simulink model "PID_Continous_Discrete"  (R2024a)
settings: Solver=FixedStepDiscrete  StartTime=0.0  StopTime=10.0  FixedStep=1e-3  RelTol=1e-3
libraries: simulink x1
settings Model: Creator=VICTUS  LastModifiedBy=VICTUS

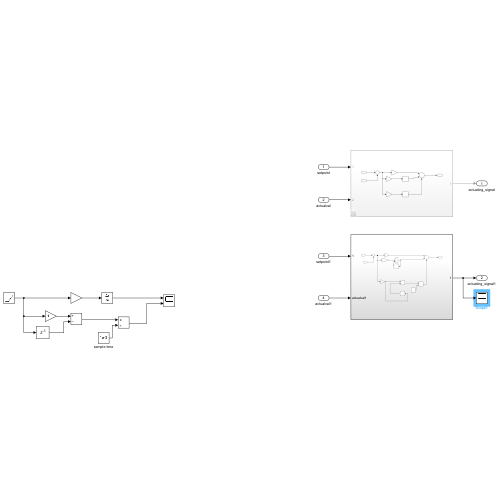
[thumbnail: Simulink's stored preview of the top-level diagram]
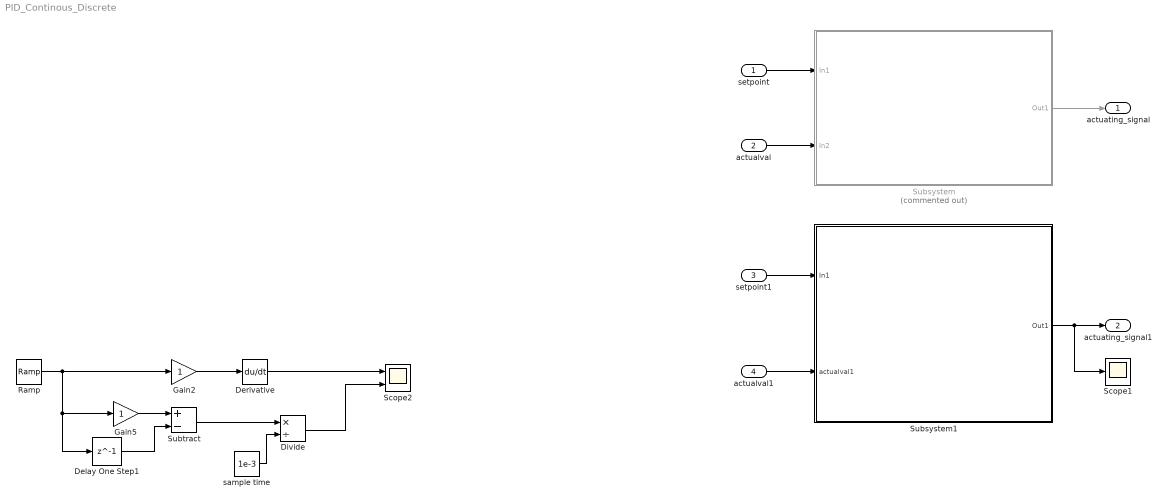
== system PID_Continous_Discrete ==
  setpoint : Inport
  actualval : Inport  Port=2
  setpoint1 : Inport  Port=3
  actualval1 : Inport  Port=4
  Delay One Step1 : Delay  DelayLength=1
  Derivative : Derivative  CoefficientInTFapproximation=1/(1e-3)
  Divide : Product  Inputs=*/
  Gain2 : Gain
  Gain5 : Gain
  Ramp : simulink/Sources/Ramp  slope=1  start=0  InitialOutput=0
  Scope1 : Scope
  Scope2 : Scope  NumInputPorts=2
  Subsystem : Subsystem  Commented=on
  Subsystem1 : Subsystem
  Subtract : Sum  Inputs=+-
  sample time : Constant  Value=1e-3
  actuating_signal : Outport
  actuating_signal1 : Outport  Port=2
  wires:
  Subsystem/1(Out1) -> actuating_signal/1
  Subsystem1/1(Out1) -> Scope1/1, actuating_signal1/1
  setpoint/1 -> Subsystem/1(In1)
  actualval/1 -> Subsystem/2(In2)
  setpoint1/1 -> Subsystem1/1(In1)
  Gain5/1 -> Subtract/1
  Delay One Step1/1 -> Subtract/2
  sample time/1 -> Divide/2
  Subtract/1 -> Divide/1
  Ramp/1 -> Gain2/1, Gain5/1, Delay One Step1/1
  Gain2/1 -> Derivative/1
  Derivative/1 -> Scope2/1
  Divide/1 -> Scope2/2
  actualval1/1 -> Subsystem1/2(actualval1)

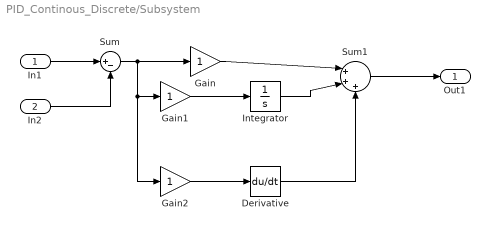
== system PID_Continous_Discrete/Subsystem ==
  In1 : Inport
  In2 : Inport  Port=2
  Derivative : Derivative
  Gain : Gain
  Gain1 : Gain
  Gain2 : Gain
  Integrator : Integrator
  Sum : Sum  Inputs=|+-
  Sum1 : Sum  Inputs=|+++
  Out1 : Outport
  wires:
  Gain1/1 -> Integrator/1
  Derivative/1 -> Sum1/3
  Sum/1 -> Gain2/1, Gain1/1, Gain/1
  Integrator/1 -> Sum1/2
  Gain2/1 -> Derivative/1
  Gain/1 -> Sum1/1
  In1/1 -> Sum/1
  Sum1/1 -> Out1/1
  In2/1 -> Sum/2

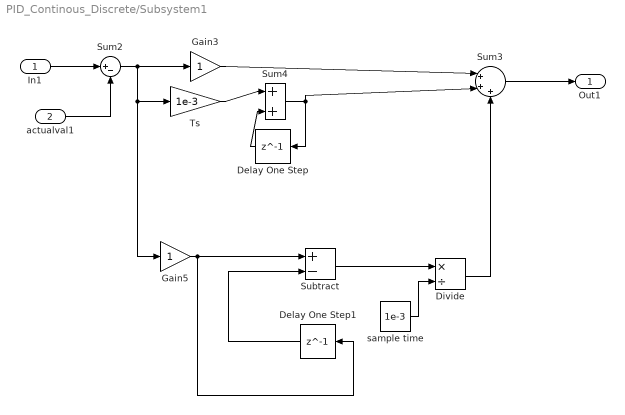
== system PID_Continous_Discrete/Subsystem1 ==
  In1 : Inport
  actualval1 : Inport  Port=2
  Delay One Step : Delay  DelayLength=1
  Delay One Step1 : Delay  DelayLength=1
  Divide : Product  Inputs=*/
  Gain3 : Gain
  Gain5 : Gain
  Subtract : Sum  Inputs=+-
  Sum2 : Sum  Inputs=|+-
  Sum3 : Sum  Inputs=|+++
  Sum4 : Sum  Inputs=|++
  Ts : Gain  Gain=1e-3
  sample time : Constant  Value=1e-3
  Out1 : Outport
  wires:
  Sum4/1 -> Sum3/2, Delay One Step/1
  Gain5/1 -> Delay One Step1/1, Subtract/1
  sample time/1 -> Divide/2
  Subtract/1 -> Divide/1
  Gain3/1 -> Sum3/1
  Delay One Step1/1 -> Subtract/2
  actualval1/1 -> Sum2/2
  Sum2/1 -> Gain3/1, Ts/1, Gain5/1
  Ts/1 -> Sum4/1
  Delay One Step/1 -> Sum4/2
  Sum3/1 -> Out1/1
  Divide/1 -> Sum3/3
  In1/1 -> Sum2/1
